simulink model "param_fcn"  (R2013a)
settings: Solver=ode45  StartTime=0.0  StopTime=10.0  RelTol=1e-3
settings Model: Creator=Maik  LastModifiedBy=Maik

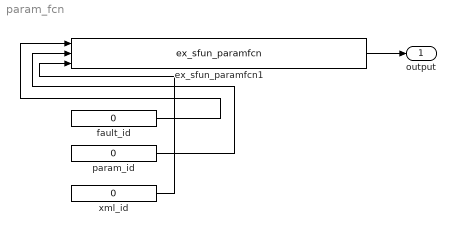
== system param_fcn ==
  ex_sfun_paramfcn1 : S-Function  FunctionName=ex_sfun_paramfcn  EnableBusSupport=off  mask(Legacy Function){SFunctionSpec=double y1 = param_fcn(single u1, single u2, single u3), ShowSpec=on}
      mask prompts: ShowSpec "Display function specification"
      mask help:
      | This block allows you to call the legacy functions specified by the following Legacy Code Tool definition:
      | def.SFunctionName = 'ex_sfun_paramfcn';
      | def.OutputFcnSpec = 'double y1 = param_fcn(single u1, single u2, single u3)';
      | def.HeaderFiles = {'param_fcn.hpp'};
      | def.SourceFiles = {'param_fcn.cpp'};
      | def.Options.language = 'C++';
      mask Help: <p>This block was generated automatically by the Legacy Code Tool. For detailed help on this tool, call<a href="matlab:legacy_code('help')"> legacy_code('help')</a>.</p>
      mask Callback ShowSpec:
      | if strcmp(get_param(gcbh, 'ShowSpec'), 'on')
      |   set_param(gcbh, 'MaskDisplay', sprintf('fprintf(''%s'');', get_param(gcbh, 'SFunctionSpec')));
      | else
      |   set_param(gcbh, 'MaskDisplay', sprintf('fprintf(''%s'');', get_param(gcbh, 'FunctionName')));
      | end
      mask Display: fprintf('%s','double y1 = param_fcn(single u1, single u2, single u3)');
  "fault_id " : Constant  Value=0  OutDataTypeStr=single
  "param_id " : Constant  Value=0  OutDataTypeStr=single
  "xml_id " : Constant  Value=0  OutDataTypeStr=single
  output : Outport
  wires:
  "fault_id "/1 -> ex_sfun_paramfcn1/1
  "param_id "/1 -> ex_sfun_paramfcn1/2
  ex_sfun_paramfcn1/1 -> output/1
  "xml_id "/1 -> ex_sfun_paramfcn1/3
